simulink library "patterns_library"  (R2014a)
settings: Solver=ode45  StartTime=0.0  StopTime=10.0  RelTol=1e-3
settings Model: Creator=lgwagner  LastModifiedBy=lgwagner

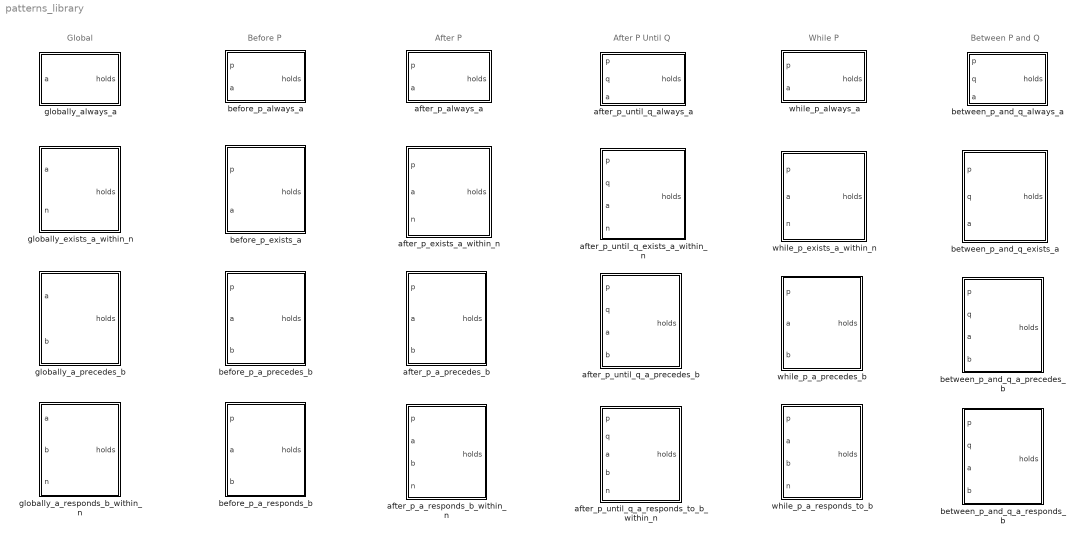
== system patterns_library ==
  note: Before P
  note: Global
  note: After P
  note: After P Until Q
  note: While P
  note: Between P and Q
  after_p_a_precedes_b : Stateflow chart  TreatAsAtomicUnit=on
  after_p_a_responds_b_within_n : Stateflow chart  TreatAsAtomicUnit=on
  after_p_always_a : Stateflow chart  TreatAsAtomicUnit=on
  after_p_exists_a_within_n : Stateflow chart  TreatAsAtomicUnit=on
  after_p_until_q_a_precedes_b : Stateflow chart  TreatAsAtomicUnit=on
  after_p_until_q_a_responds_to_b_within_n : Stateflow chart  TreatAsAtomicUnit=on
  after_p_until_q_always_a : Stateflow chart  TreatAsAtomicUnit=on
  after_p_until_q_exists_a_within_n : Stateflow chart  TreatAsAtomicUnit=on
  before_p_a_precedes_b : Stateflow chart  TreatAsAtomicUnit=on
  before_p_a_responds_b : Stateflow chart  TreatAsAtomicUnit=on
  before_p_always_a : Stateflow chart  TreatAsAtomicUnit=on
  before_p_exists_a : Stateflow chart  TreatAsAtomicUnit=on
  between_p_and_q_a_precedes_b : Stateflow chart  TreatAsAtomicUnit=on
  between_p_and_q_a_responds_b : Stateflow chart  TreatAsAtomicUnit=on
  between_p_and_q_always_a : Stateflow chart  TreatAsAtomicUnit=on
  between_p_and_q_exists_a : Stateflow chart  TreatAsAtomicUnit=on
  globally_a_precedes_b : Stateflow chart  TreatAsAtomicUnit=on
  globally_a_responds_b_within_n : Stateflow chart  TreatAsAtomicUnit=on
  globally_always_a : Stateflow chart  TreatAsAtomicUnit=on
  globally_exists_a_within_n : Stateflow chart  TreatAsAtomicUnit=on
  while_p_a_precedes_b : Stateflow chart  TreatAsAtomicUnit=on
  while_p_a_responds_to_b : Stateflow chart  TreatAsAtomicUnit=on
  while_p_always_a : Stateflow chart  TreatAsAtomicUnit=on
  while_p_exists_a_within_n : Stateflow chart  TreatAsAtomicUnit=on

== stateflow chart patterns_library/before_p_always_a ==
  settings: executeAtInitialization=1
  state state0
    en: holds=true;
  state state1
    en: holds=true;
  state state2
    en: holds=true;
  state state3
    en: holds=false;
  (default) -> state0
  state0 -> state0 [order 1] : [a && ~p]
  state0 -> state1 [order 2] : [p]
  state0 -> state2 [order 3] : [~a && ~p]
  state2 -> state3 [order 1] : [p]
  state2 -> state2 [order 2] : [~p]
  data: p input boolean; a input boolean; holds output boolean

== stateflow chart patterns_library/before_p_exists_a ==
  settings: executeAtInitialization=1
  state state0
    en: holds=true;
  state state1
    en: holds=true;
  state state2
    en: holds=false;
  (default) -> state0
  state0 -> state0 [order 1] : [~a && ~p]
  state1 -> state1
  state0 -> state1 [order 2] : [a && ~p]
  state0 -> state2 [order 3] : [p]
  state2 -> state2
  data: p input boolean; a input boolean; holds output boolean

== stateflow chart patterns_library/before_p_a_precedes_b ==
  settings: executeAtInitialization=1
  state state0
    en: holds=true;
  state state1
    en: holds=true;
  state state2
    en: holds=true;
  state state3
    en: holds=false;
  (default) -> state0
  state0 -> state0 [order 1] : [~p && ~a && ~b]
  state1 -> state1
  state0 -> state1 [order 2] : [p || a]
  state0 -> state2 [order 3] : [~p && ~a && b]
  state3 -> state3
  state2 -> state3 [order 2] : [p]
  state2 -> state2 [order 1] : [~p]
  data: p input boolean; a input boolean; holds output boolean; b input boolean

== stateflow chart patterns_library/before_p_a_responds_b ==
  settings: executeAtInitialization=1
  state state0
    en: holds=true;
  state state1
    en: holds=true;
  state state2
    en: holds=true;
  state state3
    en: holds=false;
  (default) -> state0
  state0 -> state0 [order 1] : [(~p && ~b) || (~p && a && b)]
  state1 -> state1 [order 1] : [~p && ~a]
  state0 -> state1 [order 2] : [~p && ~a && b]
  state0 -> state2 [order 3] : [p]
  state1 -> state0 [order 3] : [~p && a]
  state1 -> state3 [order 2] : [p]
  state3 -> state3
  state2 -> state2
  data: p input boolean; a input boolean; holds output boolean; b input boolean

== stateflow chart patterns_library/after_p_exists_a_within_n ==
  settings: executeAtInitialization=1
  state state0
    en: holds=true;
  state state1
    en: holds=true;
  state state3
    en: holds=false;
  state state2
    en: holds=true;
  (default) -> state0
  state1 -> state1 [order 1] : [~a && (i<n)]
  state0 -> state0 [order 1] : [~p]
  state3 -> state3
  state0 -> state1 [order 3] : [p && ~a]{i=0;}
  state1 -> state3 [order 3] : [~a && (i>=n)]
  state0 -> state2 [order 2] : [p && a]
  state1 -> state2 [order 2] : [a]
  state2 -> state2
  data: p input boolean; a input boolean; holds output boolean; i local; n input

== stateflow chart patterns_library/after_p_a_precedes_b ==
  settings: executeAtInitialization=1
  state state1
    en: holds=true;
  state state0
    en: holds=true;
  state state2
    en: holds=true;
  state state3
    en: holds=true;
  (default) -> state0
  state0 -> state0 [order 1] : [~p]
  state1 -> state1
  state0 -> state1 [order 2] : [p && a]
  state2 -> state1 [order 3] : [a]
  state0 -> state3 [order 4] : [p && ~a && b]
  state0 -> state2 [order 3] : [p && ~a && ~b]
  state2 -> state2 [order 1] : [~a && ~b]
  state2 -> state3 [order 2] : [~a && b]
  state3 -> state3
  data: p input boolean; a input boolean; holds output boolean; b input boolean

== stateflow chart patterns_library/after_p_always_a ==
  settings: executeAtInitialization=1
  state state0
    en: holds=true;
  state state1
    en: holds=true;
  state state2
    en: holds=false;
  (default) -> state0
  state0 -> state0 [order 1] : [~p]
  state1 -> state1 [order 1] : [a]
  state0 -> state1 [order 3] : [p && a]
  state0 -> state2 [order 2] : [p && ~a]
  state1 -> state2 [order 2] : [~a]
  data: p input boolean; a input boolean; holds output boolean

== stateflow chart patterns_library/after_p_a_responds_b_within_n ==
  settings: executeAtInitialization=1
  state state1
    en: holds=true;
  state state3
    en: holds=false;
  state state0
    en: holds=true;
  state state2
    en: holds=true;
  (default) -> state0
  state1 -> state1 [order 1] : [~a && (i < n)]{i = i + 1;}
  state3 -> state3
  state0 -> state0 [order 1] : [~p]
  state1 -> state3 [order 3] : [~a && (i>=n)]
  state0 -> state1 [order 2] : [p && ~a && b]{i=0;}
  state2 -> state1 [order 2] : [~a && b]
  state1 -> state2 [order 2] : [a]
  state0 -> state2 [order 3] : [(p && a) || (p && ~a && ~b)]
  state2 -> state2 [order 1] : [a || (~a && ~b)]
  data: p input boolean; a input boolean; holds output boolean; b input boolean; n input; i local

== stateflow chart patterns_library/globally_always_a ==
  settings: executeAtInitialization=1
  state state0
    en: holds=true;
  state state1
    en: holds=false;
  (default) -> state0
  state0 -> state0 [order 1] : [a]
  state1 -> state1
  state0 -> state1 [order 2] : [~a]
  data: a input boolean; holds output boolean

== stateflow chart patterns_library/globally_exists_a_within_n ==
  settings: executeAtInitialization=1
  state state0
    en: holds=true;
  state state1
    en: holds=true;
  state state2
    en: holds=false;
  (default) -> state0 : {i=0;}
  state0 -> state0 [order 1] : [~a && (i<n)]
  state1 -> state1
  state0 -> state1 [order 2] : [a]
  state0 -> state2 [order 3] : [~a && (i>=n)]
  data: a input boolean; holds output boolean; n input; i local

== stateflow chart patterns_library/globally_a_precedes_b ==
  settings: executeAtInitialization=1
  state state0
    en: holds=true;
  state state1
    en: holds=true;
  state state2
    en: holds=true;
  (default) -> state0
  state0 -> state0 [order 1] : [~a && ~b]
  state1 -> state1
  state0 -> state1 [order 2] : [a]
  state0 -> state2 [order 3] : [~a && b]
  state2 -> state2
  data: a input boolean; holds output boolean; b input boolean

== stateflow chart patterns_library/globally_a_responds_b_within_n ==
  settings: executeAtInitialization=1
  state state0
    en: holds=true;
  state state1
    en: holds=true;
  state state2
    en: holds=false;
  (default) -> state0
  state0 -> state0 [order 1] : [~b || (b && a)]
  state1 -> state1 [order 1] : [~a && (i<n)]{i = i + 1;}
  state0 -> state1 [order 2] : [b && ~a]{i=0;}
  state1 -> state1 [order 4] : [a && b]{i=0;}
  state1 -> state0 [order 3] : [~b && a]
  state1 -> state2 [order 2] : [~a && (i>=n)]
  state2 -> state2
  data: a input boolean; holds output boolean; b input boolean; n input; i local

== stateflow chart patterns_library/after_p_until_q_always_a ==
  settings: executeAtInitialization=1
  state state0
    en: holds=true;
  state state1
    en: holds=true;
  state state2
    en: holds=false;
  (default) -> state0
  state1 -> state1 [order 1] : [a && ~q]
  state0 -> state0 [order 3] : [~p || (p && q)]
  state0 -> state1 [order 1] : [p && ~q && a]
  state0 -> state2 [order 2] : [p && ~q && ~a]
  state1 -> state0 [order 2] : [q]
  state1 -> state2 [order 3] : [~a && ~q]
  data: p input boolean; q input boolean; a input boolean; holds output boolean

== stateflow chart patterns_library/after_p_until_q_exists_a_within_n ==
  settings: executeAtInitialization=1
  state state0
    en: holds=true;
  state state1
    en: holds=true;
  state state3
    en: holds=false;
  state state2
    en: holds=true;
  (default) -> state0
  state1 -> state1 [order 3] : [~q && ~a && (i < n)]{i = i + 1;}
  state0 -> state0 [order 1] : [~p || (p && q)]
  state0 -> state1 [order 2] : [p && ~q && ~a]{i=0;}
  state1 -> state3 [order 1] : [q || (~q && ~a && (i>=n))]
  state0 -> state2 [order 3] : [p && ~q && a]
  state2 -> state0 [order 3] : [q]
  state1 -> state2 [order 2] : [~q && a]
  state2 -> state1 [order 1] : [p && ~q && ~a]{i=0;}
  state2 -> state2 [order 2] : [(p && ~q && a) || (~p && ~q)]
  data: p input boolean; q input boolean; a input boolean; holds output boolean; n input; i local

== stateflow chart patterns_library/after_p_until_q_a_precedes_b ==
  settings: executeAtInitialization=1
  state state1
    en: holds=true;
  state state0
    en: holds=true;
  state state2
    en: holds=false;
  (default) -> state0
  state1 -> state1 [order 1] : [~q && ~a && ~b]
  state0 -> state1 [order 2] : [p && ~a && ~b && ~q]
  state1 -> state0 [order 2] : [q || a]
  state0 -> state0 [order 1] : [~p || (p && q) || (p && ~q && a)]
  state1 -> state2 [order 3] : [~q && ~a && b]
  state0 -> state2 [order 3] : [p && ~q && ~a && b]
  data: p input boolean; q input boolean; a input boolean; holds output boolean; b input boolean

== stateflow chart patterns_library/after_p_until_q_a_responds_to_b_within_n ==
  settings: executeAtInitialization=1
  state state0
    en: holds=true;
  state state1
    en: holds=true;
  state state2
    en: holds=true;
  state state3
    en: holds=false;
  (default) -> state0
  state0 -> state0 [order 1] : [~p || (p && q)]
  state1 -> state1 [order 2] : [(~q && q) || (~q && ~a && ~b)]
  state0 -> state1 [order 2] : [(p && ~q && a) || (p && ~q && ~a && b)]
  state1 -> state0 [order 1] : [q]
  state0 -> state2 [order 3] : [p && ~q && ~a && b]
  state1 -> state2 [order 3] : [~q && ~a && b]{i=0;}
  state2 -> state1 [order 2] : [~q && a]
  state3 -> state3
  state2 -> state3 [order 1] : [q || (~q && a && (i >=n))]
  state2 -> state2 [order 3] : [~q && ~a && (i<n)]{i = i + 1;}
  data: p input boolean; q input; a input boolean; holds output boolean; b input boolean; n input; i local

== stateflow chart patterns_library/while_p_always_a ==
  settings: executeAtInitialization=1
  state state0
    en: holds=true;
  state state2
    en: holds=false;
  (default) -> state0
  state0 -> state0 [order 1] : [~p || (p && a)]
  state0 -> state2 [order 2] : [p && ~a]
  state2 -> state2
  data: p input boolean; a input boolean; holds output boolean

== stateflow chart patterns_library/while_p_exists_a_within_n ==
  settings: executeAtInitialization=1
  state state0
    en: holds=true;
  state state1
    en: holds=true;
  state state3
    en: holds=false;
  state state2
    en: holds=true;
  (default) -> state0
  state1 -> state1 [order 2] : [p && ~a && (i < n)]{i = i + 1;}
  state0 -> state0 [order 1] : [~p]
  state3 -> state3
  state1 -> state3 [order 3] : [~p || (p && ~a && (i>=n))]
  state0 -> state1 [order 2] : [p && ~a]{i=0;}
  state2 -> state0 [order 2] : [p && a]
  state0 -> state2 [order 3] : [~p]
  state1 -> state2 [order 1] : [p && a]
  state2 -> state2 [order 1] : [p]
  data: p input boolean; a input boolean; holds output boolean; i local; n input

== stateflow chart patterns_library/while_p_a_precedes_b ==
  settings: executeAtInitialization=1
  state state0
    en: holds=true;
  state state1
    en: holds=true;
  state state2
    en: holds=true;
  (default) -> state0
  state0 -> state0 [order 1] : [~p || (p && a)]
  state1 -> state1 [order 2] : [p && ~a && ~b]
  state0 -> state1 [order 2] : [p && ~a && ~b]
  state1 -> state0 [order 1] : [~p || a]
  state0 -> state2 [order 3] : [p && ~a && b]
  state1 -> state2 [order 3] : [p && ~a && b]
  state2 -> state2
  data: p input boolean; a input boolean; holds output boolean; b input boolean

== stateflow chart patterns_library/while_p_a_responds_to_b ==
  settings: executeAtInitialization=1
  state state0
    en: holds=true;
  state state1
    en: holds=true;
  state state2
    en: holds=true;
  state state3
    en: holds=false;
  (default) -> state0
  state1 -> state1 [order 2] : [(p && a) || (p && ~a && ~b)]
  state0 -> state0 [order 1] : [~p]
  state0 -> state1 [order 2] : [(p && a) || (p && ~a && b)]
  state1 -> state0 [order 1] : [~p]
  state0 -> state2 [order 3] : [p && ~a && b]
  state1 -> state2 [order 3] : [p && ~a && b]{i=0;}
  state2 -> state1 [order 2] : [p && a]
  state3 -> state3
  state2 -> state3 [order 1] : [~p || (p && ~a && (i >= n))]
  state2 -> state2 [order 3] : [p && ~a && (i<n)]{i = i + 1;}
  data: p input boolean; a input boolean; holds output boolean; b input boolean; n input; i local

== stateflow chart patterns_library/between_p_and_q_always_a ==
  settings: executeAtInitialization=1
  state state0
    en: holds=true;
  state state1
    en: holds=true;
  state state2
    en: holds=true;
  state state3
    en: holds=false;
  (default) -> state0
  state1 -> state1 [order 2] : [~q && a]
  state0 -> state1 [order 2] : [p && ~q && a]
  state0 -> state0 [order 1] : [~p || (p && q)]
  state1 -> state0 [order 1] : [q]
  state0 -> state2 [order 3] : [p && ~q && ~a]
  state1 -> state2 [order 3] : [~q && ~a]
  state2 -> state3 [order 1] : [q]
  state3 -> state3
  state2 -> state2 [order 2] : [~q]
  data: p input boolean; q input; a input boolean; holds output boolean

== stateflow chart patterns_library/between_p_and_q_exists_a ==
  settings: executeAtInitialization=1
  state state0
    en: holds=true;
  state state1
    en: holds=true;
  state state3
    en: holds=false;
  (default) -> state0
  state1 -> state1 [order 2] : [~q && ~a]
  state0 -> state0 [order 1] : [~p || (p && a)]
  state0 -> state1 [order 2] : [p && ~a]
  state1 -> state3 [order 1] : [q]
  state1 -> state0 [order 3] : [~q && a]
  data: p input boolean; q input boolean; a input boolean; holds output boolean

== stateflow chart patterns_library/between_p_and_q_a_precedes_b ==
  settings: executeAtInitialization=1
  state state0
    en: holds=true;
  state state1
    en: holds=true;
  state state2
    en: holds=true;
  state state3
    en: holds=true;
  (default) -> state0
  state1 -> state1 [order 3] : [~a && ~b && ~q]
  state0 -> state1 [order 1] : [p && ~q && ~a && ~b]
  state0 -> state0 [order 2] : [~p || (p && q) || (p && a)]
  state1 -> state0 [order 1] : [q || a]
  state0 -> state2 [order 3] : [p && ~q && ~a && b]
  state1 -> state2 [order 2] : [~a && b && ~q]
  state2 -> state3 [order 1] : [q]
  state2 -> state2 [order 2] : [~q]
  data: p input boolean; q input boolean; a input boolean; holds output boolean; b input boolean

== stateflow chart patterns_library/between_p_and_q_a_responds_b ==
  settings: executeAtInitialization=1
  state state0
    en: holds=true;
  state state1
    en: holds=true;
  state state2
    en: holds=true;
  state state3
    en: holds=false;
  (default) -> state0
  state0 -> state0 [order 1] : [~p || (p && q)]
  state2 -> state0 [order 3] : [p && ~q && ~a && b]
  state1 -> state0 [order 2] : [q]
  state0 -> state1 [order 2] : [(p && ~q && ~b) || (p && ~q && a && b)]
  state1 -> state1 [order 3] : [(~q && a && b) || (~q && ~b)]
  state2 -> state1 [order 2] : [~q && a]
  state1 -> state2 [order 1] : [~q && ~a && b]
  state3 -> state3
  state2 -> state2 [order 4] : [~q && ~a]
  state2 -> state3 [order 1] : [q]
  data: p input boolean; q input; a input boolean; holds output boolean; b input boolean
